simulink model "ITCG_PNG_3D_salvo_simulation2"  (R2023b)
settings: Solver=ode4  StartTime=0.0  StopTime=30  FixedStep=1/10  RelTol=1e-3
libraries: simulink x4, simulink_extras x4
(part 2 of 2)

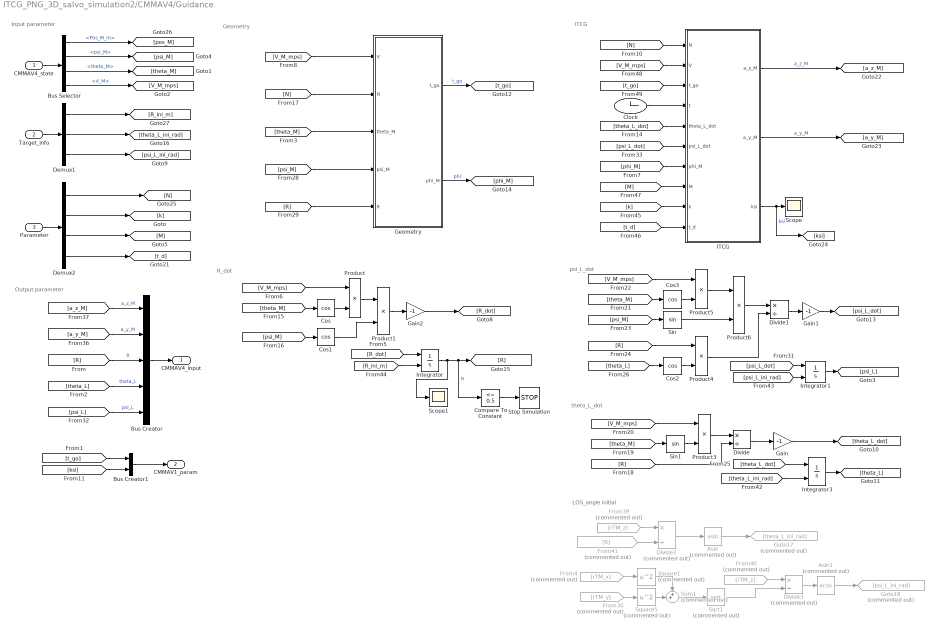
== system ITCG_PNG_3D_salvo_simulation2/CMMAV4/Guidance ==
  note: Input parameter
  note: R_dot
  note: psi_L_dot
  note: theta_L_dot
  note: LOS_angle initial
  note: Output parameter
  note: Geometry
  note: ITCG
  CMMAV4_state : Inport
  Target_info : Inport  Port=2
  Parameter : Inport  Port=3
  Asin : Trigonometry  Commented=on  Operator=asin
  Asin1 : Trigonometry  Commented=on  Operator=acos
  Bus Creator : BusCreator  Inputs=5
  Bus Creator1 : BusCreator  Inputs=2
  Bus Selector : BusSelector  OutputSignals=Pos_M_m,psi_M,theta_M,V_M
  Clock : Clock
  Compare To Constant : simulink/Logic and Bit Operations/Compare To Constant  relop=<=  const=0.5  OutDataTypeStr=boolean
  Cos{,1..3} (4 alike) : Trigonometry  Operator=cos
  Demux1 : Demux  Outputs=3
  Demux2 : Demux
  Divide : Product  Inputs=*/
  Divide1 : Product  Inputs=*/
  Divide2 : Product  Commented=on  Inputs=*/
  Divide3 : Product  Commented=on  Inputs=*/
  From30 : From  Commented=on  GotoTag=rTM_y
  From39 : From  Commented=on  GotoTag=rTM_z
  From4 : From  Commented=on  GotoTag=rTM_x
  From40 : From  Commented=on  GotoTag=rTM_z
  From41 : From  Commented=on  GotoTag=R
  Gain : Gain  Gain=-1
  Gain1 : Gain  Gain=-1
  Gain2 : Gain  Gain=-1
  Geometry : MATLAB Function  TreatAsAtomicUnit=on
  Goto17 : Goto  Commented=on  GotoTag=theta_L_ini_rad
  Goto18 : Goto  Commented=on  GotoTag=psi_L_ini_rad
  ITCG : MATLAB Function  TreatAsAtomicUnit=on
  Integrator : Integrator  InitialConditionSource=external  InitialCondition=sqrt(300^2+500^2+200^2)
  Integrator1 : Integrator  InitialConditionSource=external
  Integrator3 : Integrator  InitialConditionSource=external
  Product{,1,3..6} (6 alike) : Product
  Scope : Scope
  Scope1 : Scope
  Sin : Trigonometry
  Sin1 : Trigonometry
  Sqrt1 : Sqrt  Commented=on
  Square1 : Math  Commented=on  Operator=square
  Square5 : Math  Commented=on  Operator=square
  Stop Simulation : Stop
  Sum1 : Sum  Commented=on  Inputs=++|
  CMMAV4_input : Outport
  CMMAV1_param : Outport  Port=2
  wires:
  Product1/1 -> Gain2/1
  Gain2/1 -> [R_dot]
  [theta_L] -> Cos2/1
  [theta_L_dot] -> Integrator3/1
  Gain/1 -> [theta_L_dot]
  Product5/1 -> Product6/1
  Divide1/1 -> Gain1/1
  [V_M_mps] -> Product3/1
  [V_M_mps] -> Product5/1
  [theta_M] -> Sin1/1
  [R] -> Divide/2
  [theta_M] -> Cos3/1
  Divide/1 -> Gain/1
  [theta_M] -> Cos/1
  [R] -> Product4/1
  Product4/1 -> Divide1/2
  Integrator3/1 -> [theta_L]
  [psi_L_dot] -> Integrator1/1
  Sin1/1 -> Product3/2
  Product3/1 -> Divide/1
  [psi_M] -> Cos1/1
  Cos/1 -> Product/2
  Integrator1/1 -> [psi_L]
  Product6/1 -> Divide1/1
  [psi_M] -> Sin/1
  Compare To Constant/1 -> Stop Simulation/1
  [V_M_mps] -> Product/1
  Cos3/1 -> Product5/2
  Sin/1 -> Product6/2
  Integrator/1 -> Scope1/1, [R], Compare To Constant/1  "R"
  Product/1 -> Product1/1
  Cos2/1 -> Product4/2
  Cos1/1 -> Product1/2
  Gain1/1 -> [psi_L_dot]
  [R_dot] -> Integrator/1
  Divide3/1 -> Asin1/1
  Sum1/1 -> Sqrt1/1
  From30/1 -> Square5/1
  Square5/1 -> Sum1/2
  Square1/1 -> Sum1/1
  Asin/1 -> Goto17/1
  Sqrt1/1 -> Divide3/2
  From41/1 -> Divide2/2
  Asin1/1 -> Goto18/1
  From40/1 -> Divide3/1
  From39/1 -> Divide2/1
  From4/1 -> Square1/1
  Divide2/1 -> Asin/1
  CMMAV4_state/1 -> Bus Selector/1
  Target_info/1 -> Demux1/1
  Demux2/1 -> [N]
  Parameter/1 -> Demux2/1
  Bus Selector/1 -> [pos_M]  "<Pos_M_m>"
  Bus Selector/4 -> [V_M_mps]  "<V_M>"
  Demux1/2 -> [theta_L_ini_rad]
  Demux1/3 -> [psi_L_ini_rad]
  Demux1/1 -> [R_ini_m]
  [psi_L] -> Bus Creator/5  "psi_L"
  [theta_L] -> Bus Creator/4  "theta_L"
  Bus Creator/1 -> CMMAV4_input/1
  [a_y_M] -> Bus Creator/2  "a_y_M"
  [R] -> Bus Creator/3  "R"
  [a_z_M] -> Bus Creator/1  "a_z_M"
  [theta_L_ini_rad] -> Integrator3/2
  [psi_L_ini_rad] -> Integrator1/2
  [R_ini_m] -> Integrator/2
  Bus Selector/2 -> [psi_M]  "<psi_M>"
  Bus Selector/3 -> [theta_M]  "<theta_M>"
  Geometry/1(t_go) -> [t_go]  "t_go"
  [psi_M] -> Geometry/4(psi_M)
  Geometry/2(phi_M) -> [phi_M]  "phi"
  [V_M_mps] -> Geometry/1(V)
  [theta_M] -> Geometry/3(theta_M)
  [R] -> Geometry/5(R)
  [N] -> Geometry/2(N)
  Demux2/2 -> [k]
  Demux2/3 -> [M]
  Demux2/4 -> [t_d]
  [ksi] -> Bus Creator1/2
  [t_go] -> Bus Creator1/1
  Bus Creator1/1 -> CMMAV1_param/1
  ITCG/3(ksi) -> [ksi], Scope/1  "ksi"
  [t_d] -> ITCG/10(t_d)
  ITCG/1(a_z_M) -> [a_z_M]  "a_z_M"
  ITCG/2(a_y_M) -> [a_y_M]  "a_y_M"
  [theta_L_dot] -> ITCG/5(theta_L_dot)
  [phi_M] -> ITCG/7(phi_M)
  [t_go] -> ITCG/3(t_go)
  [N] -> ITCG/1(N)
  [M] -> ITCG/8(M)
  Clock/1 -> ITCG/4(t)
  [V_M_mps] -> ITCG/2(V)
  [k] -> ITCG/9(k)
  [psi_L_dot] -> ITCG/6(psi_L_dot)

== system ITCG_PNG_3D_salvo_simulation2/CMMAV4/Parameter init ==
  Constant : Constant  Value=3
  Constant1 : Constant  Value=2
  Constant2 : Constant  Value=10
  Constant3 : Constant  Value=30
  Mux : Mux
  Parameter : Outport
  wires:
  Mux/1 -> Parameter/1
  Constant3/1 -> Mux/4
  Constant2/1 -> Mux/3
  Constant1/1 -> Mux/2
  Constant/1 -> Mux/1

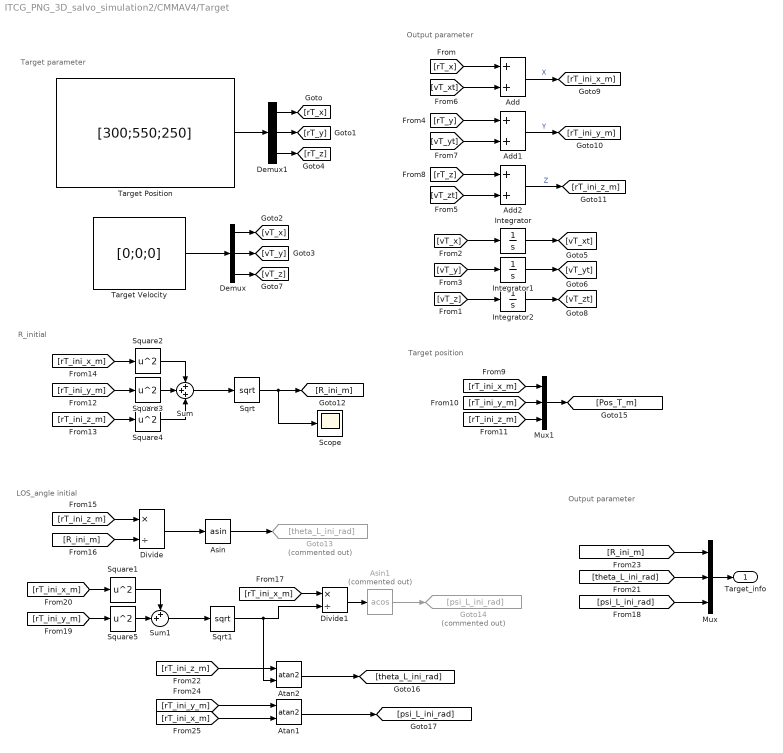
== system ITCG_PNG_3D_salvo_simulation2/CMMAV4/Target ==
  note: LOS_angle initial
  note: Target position
  note: Target parameter
  note: Output parameter
  note: R_initial
  note: Output parameter
  Add : Sum
  Add1 : Sum
  Add2 : Sum
  Asin : Trigonometry  Operator=asin
  Asin1 : Trigonometry  Commented=on  Operator=acos
  Atan1 : Trigonometry  Operator=atan2
  Atan2 : Trigonometry  Operator=atan2
  Demux : Demux  Outputs=3
  Demux1 : Demux  Outputs=3
  Divide : Product  Inputs=*/
  Divide1 : Product  Inputs=*/
  Goto13 : Goto  Commented=on  GotoTag=theta_L_ini_rad
  Goto14 : Goto  Commented=on  GotoTag=psi_L_ini_rad
  Integrator : Integrator
  Integrator1 : Integrator
  Integrator2 : Integrator
  Mux : Mux  Inputs=3
  Mux1 : Mux  Inputs=3
  Scope : Scope
  Sqrt : Sqrt
  Sqrt1 : Sqrt
  Square{1..5} (5 alike) : Math  Operator=square
  Sum : Sum  Inputs=+++
  Sum1 : Sum  Inputs=++|
  Target Position : Constant  Value=[300;550;250]  VectorParams1D=off
  Target Velocity : Constant  Value=[0;0;0]  VectorParams1D=off
  Target_info : Outport
  wires:
  [psi_L_ini_rad] -> Mux/3
  Asin/1 -> Goto13/1
  [rT_ini_z_m] -> Mux1/3
  [rT_z] -> Add2/1
  Demux/3 -> [vT_z]
  [vT_z] -> Integrator2/1
  Demux/2 -> [vT_y]
  [rT_ini_x_m] -> Mux1/1
  Add1/1 -> [rT_ini_y_m]  "Y"
  Square2/1 -> Sum/1
  [vT_x] -> Integrator/1
  Mux1/1 -> [Pos_T_m]
  Square3/1 -> Sum/2
  Add2/1 -> [rT_ini_z_m]  "Z"
  Target Position/1 -> Demux1/1
  Integrator/1 -> [vT_xt]
  Sum/1 -> Sqrt/1
  Demux1/3 -> [rT_z]
  [rT_ini_y_m] -> Mux1/2
  Integrator1/1 -> [vT_yt]
  Demux/1 -> [vT_x]
  Demux1/1 -> [rT_x]
  Target Velocity/1 -> Demux/1
  Demux1/2 -> [rT_y]
  Add/1 -> [rT_ini_x_m]  "X"
  [vT_yt] -> Add1/2
  Divide1/1 -> Asin1/1
  [rT_x] -> Add/1
  [vT_zt] -> Add2/2
  Sum1/1 -> Sqrt1/1
  [rT_ini_x_m] -> Square1/1
  Square1/1 -> Sum1/1
  Square5/1 -> Sum1/2
  [rT_ini_y_m] -> Square5/1
  [vT_y] -> Integrator1/1
  [rT_y] -> Add1/1
  [rT_ini_x_m] -> Square2/1
  [rT_ini_z_m] -> Divide/1
  [R_ini_m] -> Mux/1
  Sqrt/1 -> Scope/1, [R_ini_m]
  [R_ini_m] -> Divide/2
  [rT_ini_z_m] -> Square4/1
  [rT_ini_y_m] -> Square3/1
  [vT_xt] -> Add/2
  Divide/1 -> Asin/1
  Integrator2/1 -> [vT_zt]
  Square4/1 -> Sum/3
  [rT_ini_x_m] -> Divide1/1
  [theta_L_ini_rad] -> Mux/2
  Asin1/1 -> Goto14/1
  Mux/1 -> Target_info/1
  Sqrt1/1 -> Atan2/2, Divide1/2
  Atan2/1 -> [theta_L_ini_rad]
  [rT_ini_z_m] -> Atan2/1
  Atan1/1 -> [psi_L_ini_rad]
  [rT_ini_x_m] -> Atan1/2
  [rT_ini_y_m] -> Atan1/1

== matlab function ITCG_PNG_3D_salvo_simulation2/CMMAV1/Guidance/Geometry ==
  data: V input; N input; t_go output; phi_M output; theta_M input; psi_M input; R input
function [t_go, phi_M] =fcn(V, N, theta_M, psi_M, R)
    D2R=pi/180;

    phi_M=acos(cos(theta_M)*cos(psi_M));
    %% t_go calculate
%     a = 1 / (2 * (N - 1));
%     b = 1 / 2;
%     B1 = integral(@(t) t.^(a-1) .* (1-t).^(b-1), 0, sin(phi_M)^2, "AbsTol", 1e-6, "RelTol", 1e-4);
%     B2 = integral(@(t) t.^(a-1) .* (1-t).^(b-1), 0, 1, "AbsTol", 1e-6, "RelTol", 1e-4);
% % B1 = integral(@(t) t.^(a-1) .* (1-t).^(b-1), 0, sin(phi_M)^2);
%     B2 = integral(@(t) t.^(a-1) .* (1-t).^(b-1), 0, 1);
    % B2 = beta(a, b);

    % if isnan(B1)
    %     B1 = 0;
    % end
    % if isnan(B2)
    %     B2 = 0;
    % end

    % if abs(phi_M) >= 0 && abs(phi_M) < pi / 2
    %     t_go = (R  / (2 * V * (N-1) * sin(phi_M)^(1 / (N-1) ) ) ) * B1;
    %     if isinf(t_go)
    %         t_go = 0;
    %     end
    % 
    % else
    %     t_go = (R / (2 * V  * (N-1) * sin(phi_M)^(1 / (N-1) ) ) ) * (2 * B2 - B1);
    %     if isinf(t_go)
    %         t_go = 0;
    %     end
    % end

    t_go=(R / V) * (1 + (phi_M^2 / ( 2 * (2 * N - 1) ) ) );

== matlab function ITCG_PNG_3D_salvo_simulation2/CMMAV2/Guidance/ITCG ==
  data: a_z_M output; a_y_M output; N input; V input; t_go input; t input; theta_L_dot input; psi_L_dot input; ksi output; phi_M input; M input; k input; t_d input
function [a_z_M, a_y_M, ksi]  = fcn(N, V, t_go, t, theta_L_dot, psi_L_dot, phi_M, M, k, t_d)
    
    ksi=t_go-t_d+t;

    sgmf_ksi = 2 * ( (1 / ( 1 + exp( -10 * ksi) ) ) - 1 / 2 );
    sgmf_phi =  2 * ( (1 / ( 1 + exp( -10 * abs(phi_M) ) ) ) - 1 / 2 );
    %% Lateral ITCG command
    a_y_M = N*(1+k*sgmf_ksi)*V*psi_L_dot + M * (sgmf_phi - 1) * sgmf_ksi;

    %% Longitudinal command
    a_z_M = N * V * theta_L_dot;
    end

== matlab function ITCG_PNG_3D_salvo_simulation2/CMMAV3/Guidance/ITCG ==
  data: a_z_M output; a_y_M output; N input; V input; t_go input; t input; theta_L_dot input; psi_L_dot input; ksi output; phi_M input; M input; k input; t_d input
function [a_z_M, a_y_M, ksi]  = fcn(N, V, t_go, t, theta_L_dot, psi_L_dot, phi_M, M, k, t_d)
    
    ksi=t_go-t_d+t;

    sgmf_ksi = 2 * ( (1 / ( 1 + exp( -10 * ksi) ) ) - 1 / 2 );
    sgmf_phi =  2 * ( (1 / ( 1 + exp( -10 * abs(phi_M) ) ) ) - 1 / 2 );
    %% Lateral ITCG command
    a_y_M = N*(1+k*sgmf_ksi)*V*psi_L_dot + M * (sgmf_phi - 1) * sgmf_ksi;

    %% Longitudinal command
    a_z_M = N * V * theta_L_dot;
    end

== matlab function ITCG_PNG_3D_salvo_simulation2/CMMAV3/Guidance/Geometry ==
  data: V input; N input; t_go output; phi_M output; theta_M input; psi_M input; R input
function [t_go, phi_M] =fcn(V, N, theta_M, psi_M, R)
    D2R=pi/180;

    phi_M=acos(cos(theta_M)*cos(psi_M));
    %% t_go calculate
%     a = 1 / (2 * (N - 1));
%     b = 1 / 2;
%     B1 = integral(@(t) t.^(a-1) .* (1-t).^(b-1), 0, sin(phi_M)^2, "AbsTol", 1e-6, "RelTol", 1e-4);
%     B2 = integral(@(t) t.^(a-1) .* (1-t).^(b-1), 0, 1, "AbsTol", 1e-6, "RelTol", 1e-4);
% % B1 = integral(@(t) t.^(a-1) .* (1-t).^(b-1), 0, sin(phi_M)^2);
%     B2 = integral(@(t) t.^(a-1) .* (1-t).^(b-1), 0, 1);
    % B2 = beta(a, b);

    % if isnan(B1)
    %     B1 = 0;
    % end
    % if isnan(B2)
    %     B2 = 0;
    % end

    % if abs(phi_M) >= 0 && abs(phi_M) < pi / 2
    %     t_go = (R  / (2 * V * (N-1) * sin(phi_M)^(1 / (N-1) ) ) ) * B1;
    %     if isinf(t_go)
    %         t_go = 0;
    %     end
    % 
    % else
    %     t_go = (R / (2 * V  * (N-1) * sin(phi_M)^(1 / (N-1) ) ) ) * (2 * B2 - B1);
    %     if isinf(t_go)
    %         t_go = 0;
    %     end
    % end

    t_go=(R / V) * (1 + (phi_M^2 / ( 2 * (2 * N - 1) ) ) );

== matlab function ITCG_PNG_3D_salvo_simulation2/CMMAV4/Guidance/ITCG ==
  data: a_z_M output; a_y_M output; N input; V input; t_go input; t input; theta_L_dot input; psi_L_dot input; ksi output; phi_M input; M input; k input; t_d input
function [a_z_M, a_y_M, ksi]  = fcn(N, V, t_go, t, theta_L_dot, psi_L_dot, phi_M, M, k, t_d)
    
    ksi=t_go-t_d+t;

    sgmf_ksi = 2 * ( (1 / ( 1 + exp( -10 * ksi) ) ) - 1 / 2 );
    sgmf_phi =  2 * ( (1 / ( 1 + exp( -10 * abs(phi_M) ) ) ) - 1 / 2 );
    %% Lateral ITCG command
    a_y_M = N*(1+k*sgmf_ksi)*V*psi_L_dot + M * (sgmf_phi - 1) * sgmf_ksi;

    %% Longitudinal command
    a_z_M = N * V * theta_L_dot;
    end

== matlab function ITCG_PNG_3D_salvo_simulation2/CMMAV4/Guidance/Geometry ==
  data: V input; N input; t_go output; phi_M output; theta_M input; psi_M input; R input
function [t_go, phi_M] =fcn(V, N, theta_M, psi_M, R)
    D2R=pi/180;

    phi_M=acos(cos(theta_M)*cos(psi_M));
    %% t_go calculate
%     a = 1 / (2 * (N - 1));
%     b = 1 / 2;
%     B1 = integral(@(t) t.^(a-1) .* (1-t).^(b-1), 0, sin(phi_M)^2, "AbsTol", 1e-6, "RelTol", 1e-4);
%     B2 = integral(@(t) t.^(a-1) .* (1-t).^(b-1), 0, 1, "AbsTol", 1e-6, "RelTol", 1e-4);
% % B1 = integral(@(t) t.^(a-1) .* (1-t).^(b-1), 0, sin(phi_M)^2);
%     B2 = integral(@(t) t.^(a-1) .* (1-t).^(b-1), 0, 1);
    % B2 = beta(a, b);

    % if isnan(B1)
    %     B1 = 0;
    % end
    % if isnan(B2)
    %     B2 = 0;
    % end

    % if abs(phi_M) >= 0 && abs(phi_M) < pi / 2
    %     t_go = (R  / (2 * V * (N-1) * sin(phi_M)^(1 / (N-1) ) ) ) * B1;
    %     if isinf(t_go)
    %         t_go = 0;
    %     end
    % 
    % else
    %     t_go = (R / (2 * V  * (N-1) * sin(phi_M)^(1 / (N-1) ) ) ) * (2 * B2 - B1);
    %     if isinf(t_go)
    %         t_go = 0;
    %     end
    % end

    t_go=(R / V) * (1 + (phi_M^2 / ( 2 * (2 * N - 1) ) ) );

== matlab function ITCG_PNG_3D_salvo_simulation2/CMMAV1/Point Mass Model/MATLAB Function ==
  data: LOS_x input; NED_x output; LOS_y input; LOS_z input; psi_L input; theta_L input; NED_y output; NED_z output
function [NED_x, NED_y, NED_z] = fcn(LOS_x, LOS_y, LOS_z, psi_L, theta_L)

% 입력 벡터 (LOS 기준)
v_LOS = [LOS_x; LOS_y; LOS_z];

% 1. LOS → RCS 회전행렬 (T_LOS_to_RCS)
Rz_psi = [cos(psi_L),  sin(psi_L), 0;
         -sin(psi_L),  cos(psi_L), 0;
          0,           0,          1];

Ry_theta = [cos(theta_L), 0, -sin(theta_L);
            0,           1,  0;
            sin(theta_L), 0,  cos(theta_L)];

T_LOS_to_RCS = Ry_theta * Rz_psi;

% 2. RCS → NED 변환 (Z축 반전만 적용)
T_RCS_to_NED = [1, 0,  0;
                0, 1,  0;
                0, 0, -1];

% 전체 변환: LOS → RCS → NED
T_total = T_RCS_to_NED * T_LOS_to_RCS;

v_NED = T_total * v_LOS;

% 결과 추출
NED_x = v_NED(1);
NED_y = v_NED(2);
NED_z = v_NED(3);

end

== matlab function ITCG_PNG_3D_salvo_simulation2/Figure/MATLAB Function ==
  settings: updateMethod=DISCRETE
  data: CMMAV1_x input; CMMAV1_y input; CMMAV1_z input; CMMAV2_x input; CMMAV2_y input; CMMAV2_z input; CMMAV3_x input; CMMAV3_y input; CMMAV3_z input; CMMAV4_x input; CMMAV4_y input; CMMAV4_z input
function fcn(CMMAV1_x, CMMAV1_y, CMMAV1_z, CMMAV2_x, CMMAV2_y, CMMAV2_z, CMMAV3_x, CMMAV3_y, CMMAV3_z, CMMAV4_x, CMMAV4_y, CMMAV4_z)

persistent timeldx data1 data2 data3 data4 d12_hist d13_hist d14_hist d23_hist d24_hist d34_hist

if isempty(data1)
    data1=zeros(100000,3); data2=zeros(100000,3);
    data3=zeros(100000,3); data4=zeros(100000,3);
    d12_hist = zeros(100000,1); d13_hist = zeros(100000,1); d14_hist = zeros(100000,1);
    d23_hist = zeros(100000,1); d24_hist = zeros(100000,1); d34_hist = zeros(100000,1);
    timeldx=1;
end

CMMAV1 = [CMMAV1_x, CMMAV1_y, CMMAV1_z];
CMMAV2 = [CMMAV2_x, CMMAV2_y, CMMAV2_z];
CMMAV3 = [CMMAV3_x, CMMAV3_y, CMMAV3_z];
CMMAV4 = [CMMAV4_x, CMMAV4_y, CMMAV4_z];

data1(timeldx, :) = CMMAV1;
data2(timeldx, :) = CMMAV2;
data3(timeldx, :) = CMMAV3;
data4(timeldx, :) = CMMAV4;

d12_hist(timeldx) = norm(CMMAV1 - CMMAV2);
d13_hist(timeldx) = norm(CMMAV1 - CMMAV3);
d14_hist(timeldx) = norm(CMMAV1 - CMMAV4);
d23_hist(timeldx) = norm(CMMAV2 - CMMAV3);
d24_hist(timeldx) = norm(CMMAV2 - CMMAV4);
d34_hist(timeldx) = norm(CMMAV3 - CMMAV4);

% === Figure 1: 3D Trajectory ===
figure(1); clf; 
grid on; hold on; axis equal; view(3); box on;
plot3(data1(1:timeldx,1), data1(1:timeldx,2), data1(1:timeldx,3), 'r', 'LineWidth', 1.5);
plot3(data2(1:timeldx,1), data2(1:timeldx,2), data2(1:timeldx,3), 'b', 'LineWidth', 1.5);
plot3(data3(1:timeldx,1), data3(1:timeldx,2), data3(1:timeldx,3), 'g', 'LineWidth', 1.5);
plot3(data4(1:timeldx,1), data4(1:timeldx,2), data4(1:timeldx,3), 'm', 'LineWidth', 1.5);
scatter3(0, 0, 0, 100, 'k', 'o', 'filled');
scatter3(CMMAV1_x, CMMAV1_y, CMMAV1_z, 100, 'r', 's', 'filled');
scatter3(CMMAV2_x, CMMAV2_y, CMMAV2_z, 100, 'b', 'd', 'filled');
scatter3(CMMAV3_x, CMMAV3_y, CMMAV3_z, 100, 'g', '^', 'filled');
scatter3(CMMAV4_x, CMMAV4_y, CMMAV4_z, 100, 'm', 'p', 'filled');
legend({'UAV1','UAV2','UAV3','UAV4'}, 'Location', 'best', 'FontSize', 16, 'FontWeight', 'bold', 'FontAngle', 'italic');
xlabel('X (m)', 'FontSize', 16, 'FontWeight', 'bold', 'FontAngle', 'italic'); 
ylabel('Y (m)', 'FontSize', 16, 'FontWeight', 'bold', 'FontAngle', 'italic'); 
zlabel('Z (m)', 'FontSize', 16, 'FontWeight', 'bold', 'FontAngle', 'italic');
% xlim([-100 400]); ylim([-100 600]); zlim([0 400]);
set(gca, 'FontSize', 16, ...
         ...
         'FontAngle', 'italic', ...
         'FontName', 'Times New Roman');


% === Figure 2: Relative Distance ===
figure(2); clf;
hold on;
box on;
t_vec = 0.1 * (0:timeldx-1); 

% --- 상대거리 선들 ---
plot(t_vec, d12_hist(1:timeldx), 'r', 'LineWidth', 1.2);
plot(t_vec, d13_hist(1:timeldx), 'g', 'LineWidth', 1.2);
plot(t_vec, d14_hist(1:timeldx), 'b', 'LineWidth', 1.2);
plot(t_vec, d23_hist(1:timeldx), 'c', 'LineWidth', 1.2);
plot(t_vec, d24_hist(1:timeldx), 'm', 'LineWidth', 1.2);
plot(t_vec, d34_hist(1:timeldx), 'k', 'LineWidth', 1.2);

h = plot([0, 350], [10, 10], 'r--', 'LineWidth', 2);  

grid on;
xlabel('time [s]', 'FontWeight', 'bold', 'FontAngle', 'italic', 'FontSize', 16); 
ylabel('Relative distance [m]', 'FontWeight', 'bold', 'FontAngle', 'italic', 'FontSize', 16);
xlim([0, 30]); ylim([0 150]);
set(gca, 'FontSize', 16, ...
         ...
         'FontAngle', 'italic', ...
         'FontName', 'Times New Roman');

legend(h, 'd_{safety}', 'Location', 'best', ...
    'FontAngle', 'italic', 'FontSize', 16);

hold off;
timeldx = timeldx + 1;

end

== matlab function ITCG_PNG_3D_salvo_simulation2/CMMAV2/Guidance/Geometry ==
  data: V input; N input; t_go output; phi_M output; theta_M input; psi_M input; R input
function [t_go, phi_M] =fcn(V, N, theta_M, psi_M, R)
    D2R=pi/180;

    phi_M=acos(cos(theta_M)*cos(psi_M));
    %% t_go calculate
%     a = 1 / (2 * (N - 1));
%     b = 1 / 2;
%     B1 = integral(@(t) t.^(a-1) .* (1-t).^(b-1), 0, sin(phi_M)^2, "AbsTol", 1e-6, "RelTol", 1e-4);
%     B2 = integral(@(t) t.^(a-1) .* (1-t).^(b-1), 0, 1, "AbsTol", 1e-6, "RelTol", 1e-4);
% % B1 = integral(@(t) t.^(a-1) .* (1-t).^(b-1), 0, sin(phi_M)^2);
%     B2 = integral(@(t) t.^(a-1) .* (1-t).^(b-1), 0, 1);
    % B2 = beta(a, b);

    % if isnan(B1)
    %     B1 = 0;
    % end
    % if isnan(B2)
    %     B2 = 0;
    % end

    % if abs(phi_M) >= 0 && abs(phi_M) < pi / 2
    %     t_go = (R  / (2 * V * (N-1) * sin(phi_M)^(1 / (N-1) ) ) ) * B1;
    %     if isinf(t_go)
    %         t_go = 0;
    %     end
    % 
    % else
    %     t_go = (R / (2 * V  * (N-1) * sin(phi_M)^(1 / (N-1) ) ) ) * (2 * B2 - B1);
    %     if isinf(t_go)
    %         t_go = 0;
    %     end
    % end

    t_go=(R / V) * (1 + (phi_M^2 / ( 2 * (2 * N - 1) ) ) );

== matlab function ITCG_PNG_3D_salvo_simulation2/CMMAV1/Guidance/ITCG ==
  data: a_z_M output; a_y_M output; N input; V input; t_go input; t input; theta_L_dot input; psi_L_dot input; ksi output; phi_M input; M input; k input; t_d input
function [a_z_M, a_y_M, ksi]  = fcn(N, V, t_go, t, theta_L_dot, psi_L_dot, phi_M, M, k, t_d)
    
    ksi=t_go-t_d+t;

    sgmf_ksi = 2 * ( (1 / ( 1 + exp( -10 * ksi) ) ) - 1 / 2 );
    sgmf_phi =  2 * ( (1 / ( 1 + exp( -10 * abs(phi_M) ) ) ) - 1 / 2 );
    %% Lateral ITCG command
    a_y_M = N*(1+k*sgmf_ksi)*V*psi_L_dot + M * (sgmf_phi - 1) * sgmf_ksi;

    %% Longitudinal command
    a_z_M = N * V * theta_L_dot;
    end
